simulink subsystem "go_straight_2"  (R2022b)
settings: Solver=VariableStepAuto  StartTime=0.0  StopTime=10.0  RelTol=1e-3
settings Model: Creator=levic  LastModifiedBy=levic

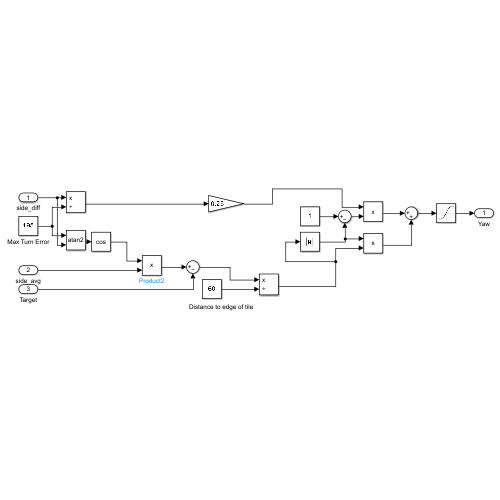
[thumbnail: Simulink's stored preview of the top-level diagram]
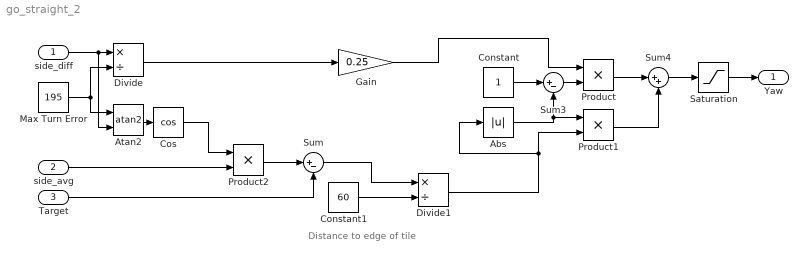
== system go_straight_2 ==
  note: Distance to edge of tile
  side_diff : Inport
  side_avg : Inport  Port=2
  Target : Inport  Port=3
  Abs : Abs  SaturateOnIntegerOverflow=off
  Atan2 : Trigonometry  Operator=atan2
  Constant : Constant
  Constant1 : Constant  Value=60
  Cos : Trigonometry  Operator=cos
  Divide : Product  Inputs=*/  RndMeth=Zero  SaturateOnIntegerOverflow=on
  Divide1 : Product  Inputs=*/  RndMeth=Zero  SaturateOnIntegerOverflow=on
  Gain : Gain  Gain=0.25
  Max Turn Error : Constant  Value=195
  Product : Product
  Product1 : Product
  Product2 : Product
  Saturation : Saturate  UpperLimit=0.25  LowerLimit=-0.25
  Sum : Sum  Inputs=|+-
  Sum3 : Sum  Inputs=|+-
  Sum4 : Sum  Inputs=|++
  Yaw : Outport
  wires:
  Target/1 -> Sum/2
  Sum3/1 -> Product/2
  Constant/1 -> Sum3/1
  Product/1 -> Sum4/1
  Product1/1 -> Sum4/2
  Sum4/1 -> Saturation/1
  Saturation/1 -> Yaw/1
  Divide1/1 -> Abs/1, Product1/2
  Abs/1 -> Sum3/2, Product1/1
  side_diff/1 -> Atan2/2, Divide/1
  Max Turn Error/1 -> Atan2/1, Divide/2
  Atan2/1 -> Cos/1
  Cos/1 -> Product2/1
  side_avg/1 -> Product2/2
  Divide/1 -> Gain/1
  Product2/1 -> Sum/1
  Sum/1 -> Divide1/1
  Gain/1 -> Product/1
  Constant1/1 -> Divide1/2
